simulink model "WindTurbineDrivelineWithVibrations"  (R2023a)
settings: Solver=ode23t  StartTime=0.0  StopTime=scenario.tEnd  MaxStep=2  RelTol=1e-3  AbsTol=1e-3
PreLoadFcn:
  | addpath('Libraries', 'Scripts_Data', 'Images');
model workspace: external: MATLAB File WindTurbineDrivelineWithVibrationsParameters.m (data not in the file)
undefined symbols (not defined in the file): Bampton, Craig, diff, fs, fsCB, m, N, rotor, scenario
libraries: fl_lib x33, nesl_utility x6, simulink x4, sdl_lib x3, slpidlib x1, nesl_utility_internal x1
(part 1 of 2)
CloseFcn:
  | clear fs hModes flex_shaft_mode_props i rotor WindTurbineOut
  | try,close(h1_sscfluids_engine_cooling_system),end
  | clear h1_sscfluids_engine_cooling_system
  | try,close(h2_sscfluids_engine_cooling_system),end
  | clear h2_WindTurbineDrivelineWithVibrations
  | try,close(h3_sscfluids_engine_cooling_system),end
  | clear h3_WindTurbineDrivelineWithVibrations
  | try,close(h4_sscfluids_engine_cooling_system),end
  | clear h4_WindTurbineDrivelineWithVibrations
  | try,close(h5_sscfluids_engine_cooling_system),end
  | clear h5_WindTurbineDrivelineWithVibrations
  | try,close(h6_sscfluids_engine_cooling_system),end
  | clear h6_WindTurbineDrivelineWithVibrations
Description:
  | Wind Turbine Driveline with Vibrations
settings Model: PauseTimes=850  LastModifiedBy=jkluger
settings SolverCC: AutoScaleAbsTol=off  SolverJacobianMethodControl=SparseAnalytical
settings DataIOCC: ReturnWorkspaceOutputsName=WindTurbineOut
settings OptimizationCC: BlockReduction=off  BooleanDataType=off  ReuseModelBlockBuffer=off
settings DebuggingCC: SaveWithParameterizedLinksMsg=none  UnderspecifiedInitializationDetection=Classic  MergeDetectMultiDrivingBlocksExec=none  SignalResolutionControl=TryResolveAllWithWarning
settings HardwareCC: TargetUnknown=on
settings ModelReferenceCC: PropagateSignalLabelsOutOfModel=off
settings SimscapeCC: SimscapeNominalValues="[{\"value\":\"1\",\"unit\":\"1/s\"},   {\"value\":\"1\",\"unit\":\"1\"}, {\"value\":\"1\",\"unit\":\"m/s\"}, {\"value\":\"1\",\"unit\":\"MW\"},{\"value\":\"10\",\"unit\":\"kN\"}, {\"value\":\"1\",\"unit\":\"cm^2\"},{\"value\":\"1\",\"unit\":\"kJ/kg\"},{\"value\":\"1\",\"unit\":\"kN*m\"},{\"value\":\"1\",\"unit\":\"V\"}]"  SimscapeLogType=all  SimscapeLogLimitData=off  SimscapeLogDataHistory=50000

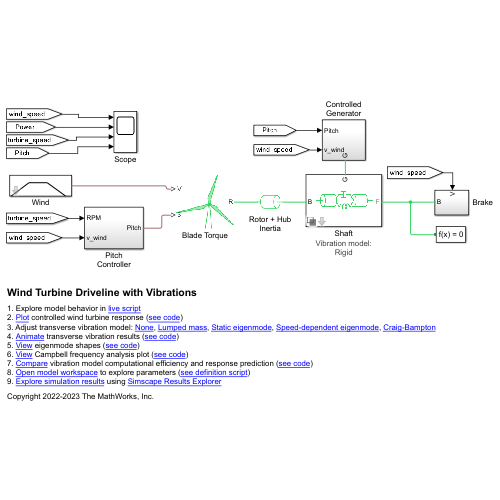
[thumbnail: Simulink's stored preview of the top-level diagram]
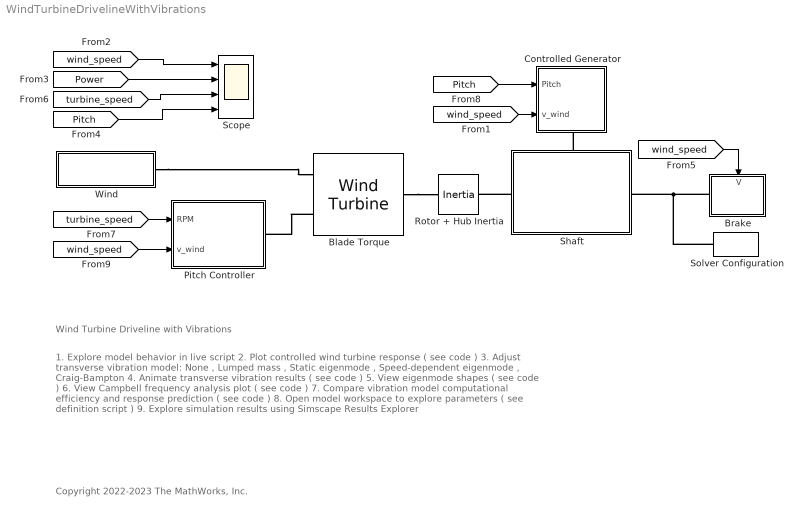
== system WindTurbineDrivelineWithVibrations ==
  note: Wind Turbine Driveline with Vibrations
  note: 1. Explore model behavior in live script
      | 2. Plot controlled wind turbine response ( see code )
      | 3. Adjust transverse vibration model: None , Lumped mass , Static eigenmode , Speed-dependent eigenmode , Craig-Bampton
      | 4. Animate transverse vibration results ( see code )
      | 5. View eigenmode shapes ( see code )
      | 6. View Campbell frequency analysis plot ( see code )
      | 7. Compare vibration model computational efficiency and response prediction ( see code )
      | 8. Open model workspace to explore parameters ( see definition script )
      | 9. Explore simulation results using Simscape Results Explorer
  note: Copyright 2022-2023 The MathWorks, Inc.
  Blade Torque : sdl_lib/Engines & Motors/Wind Turbine  model_thrust=false  R_rotor=rotor.R m  pitch_TLU=rotor.pitch deg  lambda_TLU=rotor.TSR  Cp_TLU=rotor.Cp  Ct_TLU=[0.0000, 0.2451, 0.6740, 0.9616, 1.0000, 0.9882, 0.8430, 0.0002, -0.1341; 0.0016, 0.2541, 0.5942, 0.8582, 0.9561, 0.9754, 0.9599, 0.9092, 0.8669; 0.0027, 0.2705, 0.6113, 0.8503, 0.9339, 0.9407, 0.8993, 0.8016, 0.7239; 0.0054, 0.3215, 0.6475, 0.8205, 0.8482, 0.7727, 0.5565, -0.0450, -0.1171; 0.2035, 0.4335, 0.6485, 0.6348, 0.2129, -0.1684, -0.3701, -0.5712, -0.6681; -0.05 * ones(1, 9)]  rho_air=rotor.rho kg/m^3  model_inertia=false  rotor_inertia=3.5e7 kg*m^2  init_rot_vel=0 rad/s  v_thr=0.01 m/s  w_thr=0.01 rad/s  expose_port_C=0
      settings: InternalSimscapePortConfiguration="{\"Bottom\":[],\"Left\":[{\"id\":\"vWind\",\"label\":\"V\",\"type\":\"input\"},{\"id\":\"pitch\",\"label\":\"β\",\"type\":\"input\"}],\"Right\":[{\"id\":\"R\",\"label\":\"R\",\"type\":\"foundation.mechanical.rotational.rotational\"}],\"Top\":[]}"
  Brake : Subsystem
      settings: PortSchema="{\"entries\":[{\"content\":{\"sides\":[{\"content\":{\"connectorIds\":[\"In1\"]},\"type\":\"ConnectorPlacement.EquallySpacedRectSide\",\"uuid\":\"3f522137-d01e-4a82-a213-9c95e4c48aac\"},{\"content\":{\"connectorIds\":[],\"side\":\"RIGHT\"},\"type\":\"ConnectorPlacement.EquallySpacedRectSide\",\"uuid\":\"7caeb8ed-f130-4046-b756-a57dc180120b\"},{\"content\":{\"connectorIds\":[],\"side\":\"TOP\"},\"type\":\"ConnectorPlacement.EquallySpacedRectSide\",\"uuid\":\"145b1ded-57d7-4746-892b-193b4140ae70\"},{\"content\":{\"connectorIds\":[\"RConn1\"],\"side\":\"BOTTOM\"},\"type\":\"ConnectorPlacement.EquallySpacedRectSide\",\"uuid\":\"4de12456-1f8b-4b22-93b2-a1fd618e5c7f\"}]},\"type\":\"ConnectorPlacement.EquallySpacedConnector\",\"uuid\":\"277f877b-4022-4fd4-aa9a-e474706e0074\"}],\"packageUris\":[\"http://schema.mathworks.com/mf0/Connector/R2020b\"],\"version\":\"1.0\"}"
  Controlled Generator : Subsystem
      settings: PortSchema="{\"entries\":[{\"content\":{\"sides\":[{\"content\":{\"connectorIds\":[\"In1\",\"In2\"]},\"type\":\"ConnectorPlacement.EquallySpacedRectSide\",\"uuid\":\"fea069ae-2c9f-4eba-9b7d-ddf8ed3fb909\"},{\"content\":{\"connectorIds\":[],\"side\":\"RIGHT\"},\"type\":\"ConnectorPlacement.EquallySpacedRectSide\",\"uuid\":\"deeafaeb-3537-4478-830e-60cb40e0f351\"},{\"content\":{\"connectorIds\":[],\"side\":\"TOP\"},\"type\":\"ConnectorPlacement.EquallySpacedRectSide\",\"uuid\":\"3fe5b5b4-073a-4e0c-8561-e9af00445e54\"},{\"content\":{\"connectorIds\":[\"RConn1\"],\"side\":\"BOTTOM\"},\"type\":\"ConnectorPlacement.EquallySpacedRectSide\",\"uuid\":\"d9f3141a-c426-4d0e-bc7d-6e0495890c18\"}]},\"type\":\"ConnectorPlacement.EquallySpacedConnector\",\"uuid\":\"84cb3cad-1caa-4459-9e43-abce1fcb8e5a\"}],\"packageUris\":[\"http://schema.mathworks.com/mf0/Connector/R2020b\"],\"version\":\"1.0\"}"
  Pitch Controller : Subsystem
  Rotor + Hub Inertia : fl_lib/Mechanical/Rotational Elements/Inertia  inertia=rotor.Ip_rotor_hub kg*m^2  num_ports=foundation.enum.numPorts2.two  w_specify=off  w_priority=High  w=0 rad/s  w_nominal_specify=off  w_nominal_unit=rad/s  w_nominal_value=1  t_specify=off  t_priority=None  t=0 N*m  t_nominal_specify=off  t_nominal_unit=N*m  t_nominal_value=1
      settings: InternalSimscapePortConfiguration="{\"Bottom\":[],\"Left\":[{\"id\":\"I\",\"label\":\"\",\"type\":\"foundation.mechanical.rotational.rotational\"}],\"Right\":[{\"id\":\"J\",\"label\":\"\",\"type\":\"foundation.mechanical.rotational.rotational\"}],\"Top\":[]}"
  Scope : Scope  NumInputPorts=4
  Shaft : Subsystem  Variant=on  VariantControlMode=label  VariantControl=Choice  LabelModeActiveChoice=Rigid  mask{vibration_model=Rigid, z_shaft=[0   1   2   3   4   5   6   7   8   9  10], num_modes_eig=24, num_modes_CB=8}
      mask prompts: vibration_model "Vibration model"; z_shaft "Node axial locations"; num_modes_eig "Number of eigenmodes"; num_modes_CB "Number of Craig-Bampton inner modes"
      mask init:
      | % Update num_el_lumped, num_modes_eig, or num_modes_CB
      |     vibration_model= get_param(gcb, 'vibration_model');
      |     set_param(gcb, 'vibration_model', vibration_model);
      settings: PortSchema="{\"entries\":[{\"content\":{\"sides\":[{\"content\":{\"connectorIds\":[\"LConn1\"]},\"type\":\"ConnectorPlacement.EquallySpacedRectSide\",\"uuid\":\"95241633-51a4-426a-b331-3f7eead93793\"},{\"content\":{\"connectorIds\":[\"RConn1\"],\"side\":\"RIGHT\"},\"type\":\"ConnectorPlacement.EquallySpacedRectSide\",\"uuid\":\"d2d9bb5e-ebe8-48ca-b59b-2a6070cc2ba6\"},{\"content\":{\"connectorIds\":[\"LConn2\"],\"side\":\"TOP\"},\"type\":\"ConnectorPlacement.EquallySpacedRectSide\",\"uuid\":\"f68bffd7-2afd-416e-a423-a3b5a698f394\"}]},\"type\":\"ConnectorPlacement.EquallySpacedConnector\",\"uuid\":\"6b30de51-2f46-41e0-9835-7695d3df1ab9\"}],\"packageUris\":[\"http://schema.mathworks.com/mf0/Connector/R2020b\"],\"version\":\"1.0\"}"
      settings: AttributesFormatString=|
      | Vibration model:
      | %<vibration_model>
      mask TypeOptions vibration_model: Rigid | Lumped mass | Static eigenmodes | Speed-dependent eigenmodes | Craig-Bampton
      mask Callback vibration_model:
      | vibration_model= get_param(gcb, 'vibration_model');
      |     mdlWks = get_param(bdroot,'ModelWorkspace');
      |     solver= getVariable(mdlWks, 'solver');
      |     fs= getVariable(mdlWks, 'fs');
      |     if strcmp(vibration_model, 'Rigid')
      |         paramVisibility= {'on','off', 'off', 'off'};
      |         set_param(bdroot, 'SimscapeNominalValues', solver.SimscapeNominalValues.rigid);
      |     elseif strcmp(vibration_model, 'Lumped mass')
      |         paramVisibility= {'on', 'on', 'off', 'off'};
      |         set_param(bdroot, 'SimscapeNominalValues', solver.SimscapeNominalValues.lumped_mass);
      |         z_shaft= eval(get_param(gcb, 'z_shaft'));
      |         fs.z_shaft= z_shaft;
      |         mdlWks.assignin('fs', fs)
      |     elseif strcmp(vibration_model, 'Static eigenmodes')
      |         paramVisibility= {'on', 'off', 'on', 'off'};
      |         set_param(bdroot, 'SimscapeNominalValues', solver.SimscapeNominalValues.static_eig);
      |         num_modes_eig= eval(get_param(gcb, 'num_modes_eig'));
      |         fs.num_modes= num_modes_eig;
      |         mdlWks.assignin('fs', fs);
      |     elseif strcmp(vibration_model, 'Speed-dependent eigenmodes')
      |         paramVisibility= {'on', 'off', 'on', 'off'};
      |         set_param(bdroot, 'SimscapeNominalValues', solver.SimscapeNominalValues.speed_dep_eig);
      |         num_modes_eig= eval(get_param(gcb, 'num_modes_eig'));
      |         fs.num_modes= num_modes_eig;
      |         mdlWks.assignin('fs', fs);
      |     else % vibration_model == 'Craig-Bampton'
      |         paramVisibility= {'on', 'off', 'off', 'on'};
      |         set_param(bdroot, 'SimscapeNominalValues', solver.SimscapeNominalValues.CB);
      |         fs.ne_Lumped= 50;
      |         fs.z_shaft= linspace(0, fs.length_shaft, fs.ne_Lumped);
      |         fsCB= fs;
      |         fsCB.num_modes= eval(get_param(gcb, 'num_modes_CB'));
      |         fsCB= WindTurbineDrivelineWithVibrationsCraigBamptonReduction(fsCB);
      |         mdlWks.assignin('fsCB', fsCB)
      |     end
      |     assignin('base', 'fs', fs);
      |     set_param(gcb,'MaskVisibilities',paramVisibility);
      |     set_param(gcb,'OverrideUsingVariant', vibration_model);
      mask Callback z_shaft:
      | mdlWks = get_param(bdroot,'ModelWorkspace');
      |     fs= getVariable(mdlWks, 'fs');
      |     z_shaft= eval(get_param(gcb, 'z_shaft'));
      |     fs.z_shaft= z_shaft;
      |     mdlWks = get_param(bdroot,'ModelWorkspace');
      |     mdlWks.assignin('fs', fs)
      |     assignin('base', 'fs', fs);
      mask Callback num_modes_eig:
      | mdlWks = get_param(bdroot,'ModelWorkspace');
      |     fs= getVariable(mdlWks, 'fs');
      |     num_modes_eig= eval(get_param(gcb, 'num_modes_eig'));
      |     fs.num_modes= num_modes_eig;
      |     mdlWks.assignin('fs', fs);
      |     assignin('base', 'fs', fs);
      mask Callback num_modes_CB:
      | mdlWks = get_param(bdroot,'ModelWorkspace');
      |     fs= getVariable(mdlWks, 'fs');
      |     fs.ne_Lumped= 50;
      |     fs.z_shaft= linspace(0, fs.length_shaft, fs.ne_Lumped);
      |     fsCB= fs;
      |     fsCB.num_modes= eval(get_param(gcb, 'num_modes_CB'));
      |     fsCB= WindTurbineDrivelineWithVibrationsCraigBamptonReduction(fsCB);
      |     mdlWks.assignin('fsCB', fsCB)
      |     assignin('base', 'fs', fs);
      mask DialogControl Shaft Prompt: Shaft
      mask DialogControl DescTextVar Prompt: This block models the transverse vibrations of a rotating shaft.
      mask Display: image('WindTurbineDrivelineWithVibrationsIcon.jpg');
  Solver Configuration : nesl_utility_internal/Solver Configuration  PhysicalDomain=network_engine_domain  SubClassName=solver  LeftPortType=input  RightPortType=generic  Tones=[]  Harmonics=[]  SimulateNoise=off  Profile=off  UseLocalSampling=off  EnableSwitchedLinearOptims=on  FrequencyDomain=off  UseCCode=off  RelTol=0.001  AbsTol=1e-06  MinStep=1e-09  ToWorkspace=off  RevertToSquareIcSolve=off  NumHomotopyIterations=100  PhasorMode=off  PhasorModeNumHarmonics=1  ConsistencySolver=NEWTON_XTOL_AFTER_FTOL  IndexReductionMethod=DerivativeReplacement  DoDC=off  ResidualTolerance=1e-9  ConsistencyTolSource=GLOBAL  ConsistencyAbsTol=0.001  ConsistencyRelTol=0.001  ConsistencyTolFactor=0.001  UseLocalSolver=off  LocalSolverChoice=NE_TRAPEZOIDAL_ADVANCER  ResolveIndetEquations=on  FunctionEvalNumThread=1  LocalSolverSampleTime=.002  DoFixedCost=off  MaxNonlinIter=3  MaxModeIter=2  ComputeImpulses=off  ImpulseIterations=2  LinearAlgebra=auto  LinearAlgebraNumThread=0  EquationFormulation=NE_TIME_EF  DelaysMemoryBudget=1024  AutomaticFiltering=on  FilteringTimeConstant=0.001  PartitionStorageMethod=AS_NEEDED  PartitionMemoryBudget=1024  PartitionMethod=FAST
  Wind : Subsystem  VariantControl=Ramp  mask{time=scenario.wind.Time, values=scenario.wind.Values}
      mask prompts: time "Time (s)"; values "Wind speed (m/s)"
      mask Display:
      | plot(0, 0)
      | plot(30, 30)
      | mdlWks = get_param(bdroot,'ModelWorkspace');
      | Time= evalin(mdlWks, get_param(gcb, 'time'));
      | windSpeed= evalin(mdlWks, get_param(gcb, 'values'));
      | plot(Time, windSpeed);
  wires:
  [wind_speed] -> Scope/1
  [turbine_speed] -> Scope/3
  [Power] -> Scope/2
  [Pitch] -> Scope/4
  [turbine_speed] -> Pitch Controller/1(RPM)
  [Pitch] -> Controlled Generator/1(Pitch)
  [wind_speed] -> Controlled Generator/2(v_wind)
  [wind_speed] -> Brake/1(V)
  [wind_speed] -> Pitch Controller/2(v_wind)
  connections:
  Brake/RConn1 -- Solver Configuration/RConn1 -- Shaft/RConn1
  Blade Torque/LConn2 -- Pitch Controller/RConn1
  Wind/RConn1 -- Blade Torque/LConn1
  Shaft/LConn1 -- Rotor + Hub Inertia/LConn1
  Shaft/LConn2 -- Controlled Generator/RConn1
  Blade Torque/RConn1 -- Rotor + Hub Inertia/RConn1

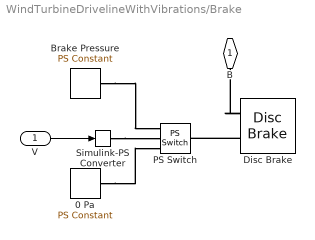
== system WindTurbineDrivelineWithVibrations/Brake ==
  V : Inport
  0 Pa : fl_lib/Physical Signals/Sources/PS Constant  constant=0 Pa
  Brake Pressure : fl_lib/Physical Signals/Sources/PS Constant  constant=10^9 Pa
  Disc Brake : sdl_lib/Brakes & Detents/Rotational/Disc Brake  r_mean=rotor.brake.radius m  bore=0.1*rotor.brake.radius m  n_pads=2  thermal_port=simscape.enum.thermaleffects.omit  mu_static=0.9  mu_coulomb=0.7  temperature_TLU=[280, 300, 320] K  mu_static_TLU=[.9, .8, .7]  mu_coulomb_TLU=[.8, .7, .6]  brkwy_vel=0.1 rad/s  visc_coef=0 N*m/(rad/s)  enable_faults=simscape.enum.onoff.off  faulted_pressure=0 bar  external_fault=simscape.enum.onoff.off  temporal_fault=simscape.enum.onoff.off  fault_time=5 s  report_fault=simscape.enum.assert.action.none  thermal_mass=50 kJ/K  temperature_specify=off  temperature_priority=High  temperature=300 K  temperature_nominal_specify=off  temperature_nominal_unit=K  temperature_nominal_value=1
  PS Switch : fl_lib/Physical Signals/Nonlinear Operators/PS Switch  Threshold=rotor.max_wind_speed m/s
      settings: InternalSimscapePortConfiguration="{\"Bottom\":[],\"Left\":[{\"id\":\"I1\",\"label\":\"\",\"type\":\"input\"},{\"id\":\"I2\",\"label\":\"\",\"type\":\"input\"},{\"id\":\"I3\",\"label\":\"\",\"type\":\"input\"}],\"Right\":[{\"id\":\"O\",\"label\":\"\",\"type\":\"output\"}],\"Top\":[]}"
  Simulink-PS Converter : nesl_utility/Simulink-PS Converter  PhysicalDomain=network_engine_domain  SubClassName=ps_input  LeftPortType=input  RightPortType=output  PseudoPeriodic=off  Frequencies=[]  NoiseDistribution=none  NoiseParameters=[]  Unit=m/s  AffineConversion=off  FilteringAndDerivatives=provide  SimscapeFilterOrder=1  InputFilterTimeConstant=0.001  UdotUserProvided=0
  B : PMIOPort  Side=Right
  wires:
  V/1 -> Simulink-PS Converter/1
  connections:
  Disc Brake/LConn2 -- B/RConn1
  Disc Brake/LConn1 -- PS Switch/RConn1
  Simulink-PS Converter/RConn1 -- PS Switch/LConn2
  0 Pa/RConn1 -- PS Switch/LConn3
  Brake Pressure/RConn1 -- PS Switch/LConn1

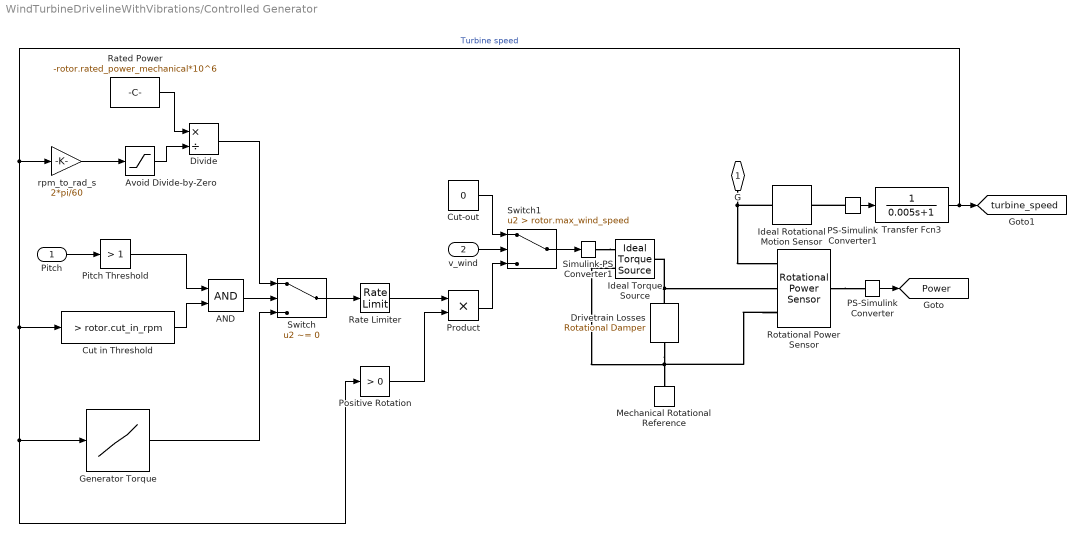
== system WindTurbineDrivelineWithVibrations/Controlled Generator ==
  Pitch : Inport
  v_wind : Inport  Port=2
  AND : Logic  AllPortsSameDT=off  OutDataTypeStr=boolean
  Avoid Divide-by-Zero : Saturate  UpperLimit=inf  LowerLimit=0.01  ZeroCross=off
  Cut in Threshold : simulink/Logic and Bit Operations/Compare To Constant  relop=>  const=rotor.cut_in_rpm  OutDataTypeStr=boolean
  Cut-out : Constant  Value=0
  Divide : Product  Inputs=*/
  Drivetrain Losses : fl_lib/Mechanical/Rotational Elements/Rotational Damper  D=rotor.drivetrain_losses_damping N*m/(rad/s)  w_specify=off  w_priority=None  w=0 rad/s  w_nominal_specify=off  w_nominal_unit=rad/s  w_nominal_value=1  t_specify=off  t_priority=None  t=0 N*m  t_nominal_specify=off  t_nominal_unit=N*m  t_nominal_value=1
  Generator Torque : Lookup_n-D  NumberOfTableDimensions=1  BreakpointsForDimension1=rotor.generator_speed_TLU % rpm  Table=-rotor.generator_torque_TLU % N*m  ExtrapMethod=Clip  UseLastTableValue=on  InternalRulePriority=Speed  RndMeth=Simplest
  Ideal Torque Source : fl_lib/Mechanical/Mechanical Sources/Ideal Torque Source
  Ideal Rotational Motion Sensor : fl_lib/Mechanical/Mechanical Sensors/Ideal Rotational Motion Sensor  reference=foundation.enum.MeasurementReference.absolute  acceleration_port=false  velocity_port=true  position_port=false  wrap_angle=simscape.enum.onoff.off  offset=0 rad
      settings: InternalSimscapePortConfiguration="{\"Bottom\":[],\"Left\":[{\"id\":\"R\",\"label\":\"R\",\"type\":\"foundation.mechanical.rotational.rotational\"}],\"Right\":[{\"id\":\"W\",\"label\":\"W\",\"type\":\"output\"}],\"Top\":[]}"
  Mechanical Rotational Reference : fl_lib/Mechanical/Rotational Elements/Mechanical Rotational Reference
  PS-Simulink Converter : nesl_utility/PS-Simulink Converter  PhysicalDomain=network_engine_domain  SubClassName=ps_output  LeftPortType=input  RightPortType=output  PseudoPeriodic=off  Frequencies=[]  VectorFormat=1-D array  Unit=MW  AffineConversion=off
  PS-Simulink Converter1 : nesl_utility/PS-Simulink Converter  PhysicalDomain=network_engine_domain  SubClassName=ps_output  LeftPortType=input  RightPortType=output  PseudoPeriodic=off  Frequencies=[]  VectorFormat=1-D array  Unit=rpm  AffineConversion=off
  Pitch Threshold : simulink/Logic and Bit Operations/Compare To Constant  relop=>  const=1  OutDataTypeStr=boolean  ZeroCross=off
  Positive Rotation : simulink/Logic and Bit Operations/Compare To Constant  relop=>  const=0  OutDataTypeStr=boolean  ZeroCross=off
  Product : Product
  Rate Limiter : RateLimiter  RisingSlewLimit=rotor.torque_rated*5  FallingSlewLimit=-rotor.torque_rated*5  SampleTimeMode=inherited
  Rated Power : Constant  Value=-rotor.rated_power_mechanical*10^6
  Rotational Power Sensor : sdl_lib/Sensors/Rotational Power Sensor  measurement_type=sdl.enum.rotationalPowerSensorType.instantaneous  averaging_period=1 s  max_frequency=1000 Hz  max_speed=1000 rpm
      settings: InternalSimscapePortConfiguration="{\"Bottom\":[],\"Left\":[{\"id\":\"S\",\"label\":\"S\",\"type\":\"foundation.mechanical.rotational.rotational\"},{\"id\":\"R\",\"label\":\"R\",\"type\":\"foundation.mechanical.rotational.rotational\"},{\"id\":\"C\",\"label\":\"C\",\"type\":\"foundation.mechanical.rotational.rotational\"}],\"Right\":[{\"id\":\"P\",\"label\":\"P\",\"type\":\"output\"}],\"Top\":[]}"
  Simulink-PS Converter1 : nesl_utility/Simulink-PS Converter  PhysicalDomain=network_engine_domain  SubClassName=ps_input  LeftPortType=input  RightPortType=output  PseudoPeriodic=off  Frequencies=[]  NoiseDistribution=none  NoiseParameters=[]  Unit=N*m  AffineConversion=off  FilteringAndDerivatives=provide  SimscapeFilterOrder=1  InputFilterTimeConstant=0.001  UdotUserProvided=0
  Switch : Switch  Criteria=u2 ~= 0  Threshold=1  SaturateOnIntegerOverflow=off  InputSameDT=off
  Switch1 : Switch  Criteria=u2 > Threshold  Threshold=rotor.max_wind_speed  SaturateOnIntegerOverflow=off  InputSameDT=off
  Transfer Fcn3 : TransferFcn  Denominator=[0.005 1]
  rpm_to_rad_s : Gain  Gain=2*pi/60
  G : PMIOPort  Side=Right
  tag scope: Power=global, turbine_speed=global
  wires:
  PS-Simulink Converter/1 -> [Power]
  Transfer Fcn3/1 -> [turbine_speed], Generator Torque/1, Positive Rotation/1, Cut in Threshold/1, rpm_to_rad_s/1  "Turbine speed"
  Switch/1 -> Rate Limiter/1
  Generator Torque/1 -> Switch/3
  Rated Power/1 -> Divide/1
  Avoid Divide-by-Zero/1 -> Divide/2
  Divide/1 -> Switch/1
  rpm_to_rad_s/1 -> Avoid Divide-by-Zero/1
  PS-Simulink Converter1/1 -> Transfer Fcn3/1
  v_wind/1 -> Switch1/2
  Cut-out/1 -> Switch1/1
  Switch1/1 -> Simulink-PS Converter1/1
  Pitch/1 -> Pitch Threshold/1
  Pitch Threshold/1 -> AND/1
  Cut in Threshold/1 -> AND/2
  AND/1 -> Switch/2
  Rate Limiter/1 -> Product/1
  Positive Rotation/1 -> Product/2
  Product/1 -> Switch1/3
  connections:
  Drivetrain Losses/LConn1 -- Rotational Power Sensor/LConn2 -- Ideal Torque Source/LConn1
  Rotational Power Sensor/LConn3 -- Drivetrain Losses/RConn1 -- Ideal Torque Source/RConn2 -- Mechanical Rotational Reference/LConn1
  Rotational Power Sensor/RConn1 -- PS-Simulink Converter/LConn1
  G/RConn1 -- Ideal Rotational Motion Sensor/LConn1 -- Rotational Power Sensor/LConn1
  Simulink-PS Converter1/RConn1 -- Ideal Torque Source/RConn1
  PS-Simulink Converter1/LConn1 -- Ideal Rotational Motion Sensor/RConn1

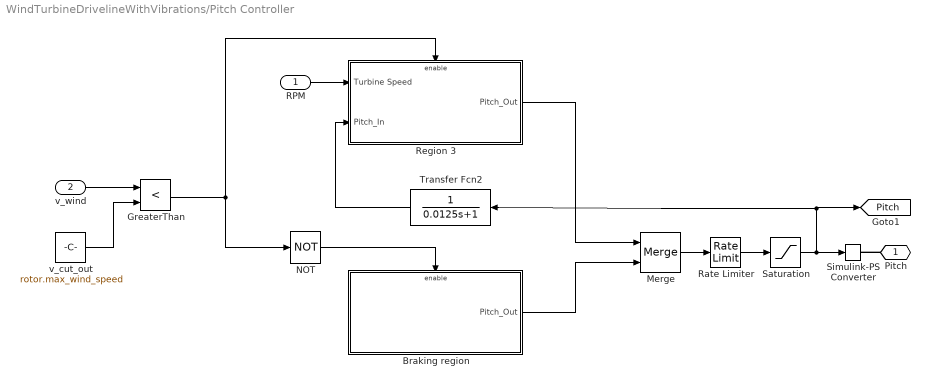
== system WindTurbineDrivelineWithVibrations/Pitch Controller ==
  RPM : Inport
  v_wind : Inport  Port=2
  Braking region : Subsystem
  GreaterThan : RelationalOperator  Operator=<  OutDataTypeStr=boolean  ZeroCross=off  RndMeth=Simplest  InputSameDT=off
  Merge : Merge
  NOT : Logic  Operator=NOT  AllPortsSameDT=off  OutDataTypeStr=boolean
  Rate Limiter : RateLimiter  RisingSlewLimit=8  FallingSlewLimit=-8  SampleTimeMode=inherited
  Region 3 : Subsystem
  Saturation : Saturate  UpperLimit=90  LowerLimit=0  ZeroCross=off
  Simulink-PS Converter : nesl_utility/Simulink-PS Converter  PhysicalDomain=network_engine_domain  SubClassName=ps_input  LeftPortType=input  RightPortType=output  PseudoPeriodic=off  Frequencies=[]  NoiseDistribution=none  NoiseParameters=[]  Unit=deg  AffineConversion=off  FilteringAndDerivatives=provide  SimscapeFilterOrder=1  InputFilterTimeConstant=0.001  UdotUserProvided=0
  Transfer Fcn2 : TransferFcn  Denominator=[0.0125 1]
  v_cut_out : Constant  Value=rotor.max_wind_speed
  Pitch : PMIOPort  Side=Right
  tag scope: Pitch=global
  wires:
  RPM/1 -> Region 3/1(Turbine Speed)
  Transfer Fcn2/1 -> Region 3/2(Pitch_In)
  Saturation/1 -> Transfer Fcn2/1, [Pitch], Simulink-PS Converter/1
  v_wind/1 -> GreaterThan/1
  v_cut_out/1 -> GreaterThan/2
  GreaterThan/1 -> NOT/1, Region 3/Enable
  Region 3/1(Pitch_Out) -> Merge/1
  Braking region/1(Pitch_Out) -> Merge/2
  Rate Limiter/1 -> Saturation/1
  Merge/1 -> Rate Limiter/1
  NOT/1 -> Braking region/Enable
  connections:
  Pitch/RConn1 -- Simulink-PS Converter/RConn1

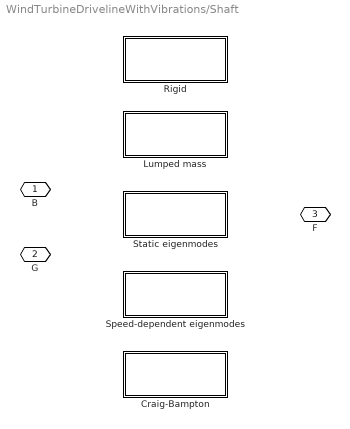
== system WindTurbineDrivelineWithVibrations/Shaft ==
  Craig-Bampton : Subsystem  VariantControl=Craig-Bampton
  Lumped mass : Subsystem  VariantControl=Lumped mass
  Rigid : Subsystem  VariantControl=Rigid
  Speed-dependent eigenmodes : Subsystem  VariantControl=Speed-dependent eigenmodes
  Static eigenmodes : Subsystem  VariantControl=Static eigenmodes
  B : PMIOPort  Side=Left
  G : PMIOPort  Port=2  Side=Left
  F : PMIOPort  Port=3  Side=Right

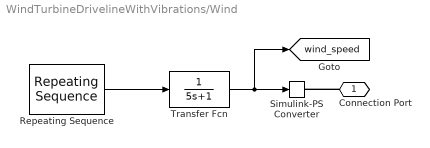
== system WindTurbineDrivelineWithVibrations/Wind ==
  Repeating Sequence : simulink/Sources/Repeating Sequence  rep_seq_t=time  rep_seq_y=values
  Simulink-PS Converter : nesl_utility/Simulink-PS Converter  PhysicalDomain=network_engine_domain  SubClassName=ps_input  LeftPortType=input  RightPortType=output  PseudoPeriodic=off  Frequencies=[]  NoiseDistribution=none  NoiseParameters=[]  Unit=m/s  AffineConversion=off  FilteringAndDerivatives=provide  SimscapeFilterOrder=1  InputFilterTimeConstant=0.001  UdotUserProvided=0
  Transfer Fcn : TransferFcn  Denominator=[5 1]
  Connection Port : PMIOPort  Side=Right
  tag scope: wind_speed=global
  wires:
  Repeating Sequence/1 -> Transfer Fcn/1
  Transfer Fcn/1 -> [wind_speed], Simulink-PS Converter/1
  connections:
  Connection Port/RConn1 -- Simulink-PS Converter/RConn1

== system WindTurbineDrivelineWithVibrations/Pitch Controller/Braking region ==
  Enable : EnablePort
  Feather Blades : Constant  Value=90
  Pitch_Out : Outport  InitialOutput=90
  wires:
  Feather Blades/1 -> Pitch_Out/1

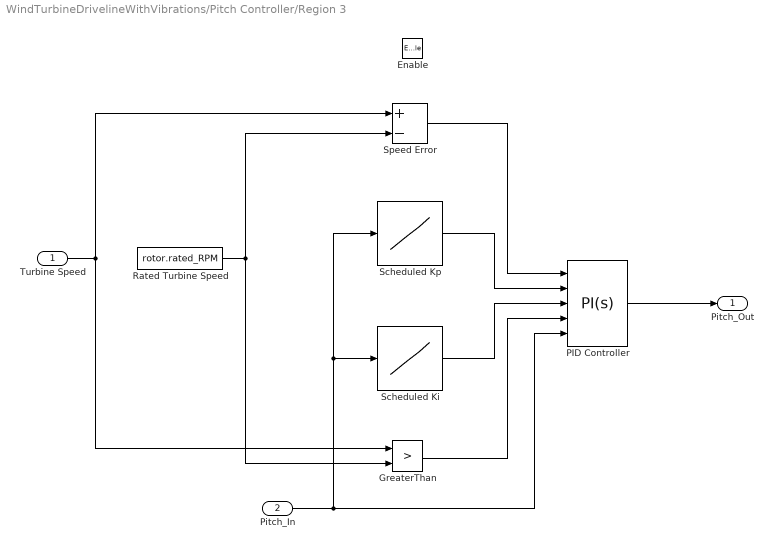
== system WindTurbineDrivelineWithVibrations/Pitch Controller/Region 3 ==
  Turbine Speed : Inport
  Pitch_In : Inport  Port=2
  Enable : EnablePort  StatesWhenEnabling=reset
  GreaterThan : RelationalOperator  Operator=>  OutDataTypeStr=boolean  ZeroCross=off  RndMeth=Simplest  InputSameDT=off
  PID Controller : slpidlib/PID Controller  Controller=PI  Form=Parallel  TimeDomain=Continuous-time  UseExternalTs=off  SampleTime=-1  IntegratorMethod=Forward Euler  FilterMethod=Forward Euler  ControllerParametersSource=external  P=0.12  I=8  UseKiTs=off  D=0  N=100  UseFilter=on  TunerSelectOption=Transfer Function Based (PID Tuner App)  ZeroCross=off  InitialConditionSource=external  InitialConditionForIntegrator=rotor.pitch(1)  InitialConditionForFilter=0  DifferentiatorICPrevScaledInput=0  ExternalReset=either  TrackingMode=off  Kt=1  LimitOutput=on  SatLimitsSource=internal  UpperSaturationLimit=90  LowerSaturationLimit=0  LinearizeAsGain=on  AntiWindupMode=none  Kb=1  LimitIntegrator=off  UpperIntegratorSaturationLimit=inf  LowerIntegratorSaturationLimit=-inf  POutMin=[]  POutMax=[]  IOutMin=[]  IOutMax=[]  DOutMin=[]  DOutMax=[]  NOutMin=[]  NOutMax=[]  SumOutMin=[]  SumOutMax=[]  SaturationOutMin=[]  SaturationOutMax=[]  PParamMin=[]  PParamMax=[]  IParamMin=[]  IParamMax=[]  DParamMin=[]  DParamMax=[]  NParamMin=[]  NParamMax=[]  KbParamMin=[]  KbParamMax=[]  KtParamMin=[]  KtParamMax=[]  KbOutMin=[]  KbOutMax=[]  KtOutMin=[]  KtOutMax=[]  IntegratorOutMin=[]  IntegratorOutMax=[]  FilterOutMin=[]  FilterOutMax=[]  SumI1OutMin=[]  SumI1OutMax=[]  SumI2OutMin=[]  SumI2OutMax=[]  SumI3OutMin=[]  SumI3OutMax=[]  SumI4OutMin=[]  SumI4OutMax=[]  SumDOutMin=[]  SumDOutMax=[]  DifferentiatorOutMin=[]  DifferentiatorOutMax=[]  FilterDiffOutCoefMin=[]  FilterDiffOutCoefMax=[]  ReciprocalOutMin=[]  ReciprocalOutMax=[]  SumDenOutMin=[]  SumDenOutMax=[]  SumNumOutMin=[]  SumNumOutMax=[]  DivideOutMin=[]  DivideOutMax=[]  UdiffTsProdOutMin=[]  UdiffTsProdOutMax=[]  NTsProdOutMin=[]  NTsProdOutMax=[]  UintegralTsProdOutMin=[]  UintegralTsProdOutMax=[]  UngainTsProdOutMin=[]  UngainTsProdOutMax=[]  ClampingZeroOutDataTypeStr=Inherit: Inherit via back propagation  ClampingZeroOutMin=[]  ClampingZeroOutMax=[]  FilterDenConstantOutDataTypeStr=Inherit: Inherit via back propagation  FilterDenConstantOutMin=[]  FilterDenConstantOutMax=[]  PCopyOutDataTypeStr=Inherit: Inherit via back propagation  PCopyOutMin=[]  PCopyOutMax=[]  NCopyOutDataTypeStr=Inherit: Inherit via back propagation  NCopyOutMin=[]  NCopyOutMax=[]  IntegratorContinuousStateAttributes=''  IntegratorStateMustResolveToSignalObject=off  IntegratorRTWStateStorageClass=Auto  FilterContinuousStateAttributes=''  FilterStateMustResolveToSignalObject=off  FilterRTWStateStorageClass=Auto  ParallelPVariant=ExternalParameters  IdealPVariant=Disabled  IVariant=ExternalParameters  DVariant=Disabled  IntegratorVariant=Continuous  SatVariant=Enabled  AWVariant=Passthrough  PCopyVariant=Disabled  TRVariant=Disabled  FdbkBlocksVariant=Forward  IdealPFdbkVariant=Disabled  SatFdbkVariant=Disabled  DerivativeFilterVariant=Disabled  NVariant=Disabled  NCopyVariant=Disabled_SignalSpec  FilterICVariant=Disabled  IntegratorICVariant=ExternalICs  ExternalResetVariant=ExternalReset  TRSumVariant=Passthrough  SumFdbkVariant=Disabled  SumVariant=Sum_PI  TsampFilterVariant=InternalTs  TsampNgainVariant=Passthrough  TsampIntegralVariant=Disabled_SignalSpec  ExternalSaturationOutDataTypeStr=Inherit: Same as second input
  Rated Turbine Speed : Constant  Value=rotor.rated_RPM
  Scheduled Ki : Lookup_n-D  NumberOfTableDimensions=1  BreakpointsForDimension1=rotor.pitch_TLU  Table=rotor.pitch_Ki_TLU  InternalRulePriority=Speed  RndMeth=Simplest
  Scheduled Kp : Lookup_n-D  NumberOfTableDimensions=1  BreakpointsForDimension1=rotor.pitch_TLU  Table=rotor.pitch_Kp_TLU  InternalRulePriority=Speed  RndMeth=Simplest
  Speed Error : Sum  Inputs=+-
  Pitch_Out : Outport
  wires:
  Pitch_In/1 -> Scheduled Ki/1, Scheduled Kp/1, PID Controller/5
  Scheduled Kp/1 -> PID Controller/2
  Speed Error/1 -> PID Controller/1
  Scheduled Ki/1 -> PID Controller/3
  Turbine Speed/1 -> GreaterThan/1, Speed Error/1
  Rated Turbine Speed/1 -> GreaterThan/2, Speed Error/2
  GreaterThan/1 -> PID Controller/4
  PID Controller/1 -> Pitch_Out/1

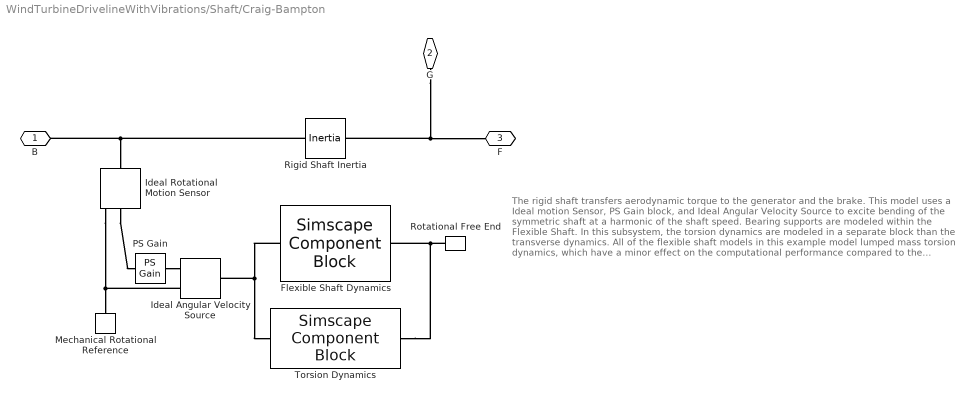
== system WindTurbineDrivelineWithVibrations/Shaft/Craig-Bampton ==
  note: The rigid shaft transfers aerodynamic torque to the generator and the brake.
      |
      | This model uses a Ideal motion Sensor, PS Gain block, and Ideal Angular Velocity Source to excite bending of the symmetric shaft at a harmonic of the shaft speed. Bearing supports are modeled within the Flexible Shaft.
      |
      | In this subsystem, the torsion dynamics are modeled in a separate block than the transverse dynamics. All of the flexible shaft models in this example model lumped mass torsion dynamics, which have a minor effect on the computational performance compared to the transverse dynamics.
  Flexible Shaft Dynamics : SimscapeComponentBlock  SourceFile=WindTurbineDrivelineWithVibrationsFlexibleShaftCB  ComponentPath=WindTurbineDrivelineWithVibrationsFlexibleShaftCB  ComponentVariants="[\"WindTurbineDrivelineWithVibrationsFlexibleShaftCB\"]"  ComponentVariantNames="[\"WindTurbineDrivelineWithVibrationsFlexibleShaftCB\"]"  ClassName=WindTurbineDrivelineWithVibrationsFlexibleShaftCB  SchemaVersion=1  M=fsCB.M  normM=fsCB.normM  G=fsCB.G  K=fsCB.K 1/s^2  alpha=fsCB.a_damp 1/s  beta=fsCB.b_damp s  ForceMagnitude=fsCB.F  num_primary_nodes=fsCB.num_primary_nodes  eta_nominal_value=solver.SimscapeNominalValues.fsCB.mode_displacements  etaDer_nominal_value=SimscapeNominalValues.fsCB.mode_velocities  support_node=fsCB.support_nodes  bearing_speed=fs.bearing_speed rad/s  K_supportB1=fs.bearing.K N/m  D_supportB1=fs.bearing.D N*s/m  Krot_supportB1=fs.bearing.k_rot N*m/rad  Drot_supportB1=fs.bearing.d_rot N*m*s/rad  K_supportI1=fs.bearing.K N/m  D_supportI1=fs.bearing.D N*s/m  Krot_supportI1=fs.bearing.k_rot N*m/rad  Drot_supportI1=fs.bearing.d_rot N*m*s/rad  K_supportI2=fs.bearing.K N/m  D_supportI2=fs.bearing.D N*s/m  Krot_supportI2=fs.bearing.k_rot N*m/rad  Drot_supportI2=fs.bearing.d_rot N*m*s/rad  K_supportI3=fs.bearing.k_trans_speed_Free N/m  D_supportI3=fs.bearing.d_trans_speed_Free N*s/m  Krot_supportI3=fs.bearing.k_rot_Free N*m/rad  Drot_supportI3=fs.bearing.d_rot_Free N*m*s/rad  K_supportF1=fs.bearing.K N/m  D_supportF1=fs.bearing.D N*s/m  Krot_supportF1=fs.bearing.k_rot N*m/rad  Drot_supportF1=fs.bearing.d_rot N*m*s/rad  t_specify=off  t_priority=None  t=0 N*m  t_nominal_specify=off  t_nominal_unit=N*m  t_nominal_value=1  w_specify=off  w_priority=None  w=0 rad/s  w_nominal_specify=off  w_nominal_unit=rad/s  w_nominal_value=1  wDer_specify=off  wDer_priority=None  wDer=0 rad/s^2  wDer_nominal_specify=off  wDer_nominal_unit=rad/s^2  wDer_nominal_value=1  phi_specify=off  phi_priority=None  phi=0 rad  phi_nominal_specify=off  phi_nominal_unit=rad  phi_nominal_value=1  Bfx_specify=off  Bfx_priority=None  Bfx=0 N  Bfx_nominal_specify=off  Bfx_nominal_unit=N  Bfx_nominal_value=1  Bfy_specify=off  Bfy_priority=None  Bfy=0 N  Bfy_nominal_specify=off  Bfy_nominal_unit=N  Bfy_nominal_value=1  BTx_specify=off  BTx_priority=None  BTx=0 N*m  BTx_nominal_specify=off  BTx_nominal_unit=N*m  BTx_nominal_value=1  BTy_specify=off  BTy_priority=None  BTy=0 N*m  BTy_nominal_specify=off  BTy_nominal_unit=N*m  BTy_nominal_value=1
      settings: CopyFcn=simscape.engine.sli.internal.componentblockcallback(gcbh,'COPY')  PreCopyFcn=simscape.engine.sli.internal.componentblockcallback(gcbh,'PRECOPY')  PreDeleteFcn=simscape.engine.sli.internal.componentblockcallback(gcbh,'PREDELETE')  InternalSimscapePortConfiguration="{\"Bottom\":[],\"Left\":[{\"id\":\"B\",\"label\":\"B\",\"type\":\"foundation.mechanical.rotational.rotational\"}],\"Right\":[{\"id\":\"F\",\"label\":\"F\",\"type\":\"foundation.mechanical.rotational.rotational\"}],\"Top\":[]}"
      mask Type: Craig-Bampton Flexible Shaft
  Ideal Angular Velocity Source : fl_lib/Mechanical/Mechanical Sources/Ideal Angular Velocity Source
  Ideal Rotational Motion Sensor : fl_lib/Mechanical/Mechanical Sensors/Ideal Rotational Motion Sensor  reference=foundation.enum.MeasurementReference.difference  acceleration_port=false  velocity_port=true  position_port=true  wrap_angle=false  offset=0 rad
  Mechanical Rotational Reference : fl_lib/Mechanical/Rotational Elements/Mechanical Rotational Reference
  PS Gain : fl_lib/Physical Signals/Functions/PS Gain  gain=fs.excitationPoles
  Rigid Shaft Inertia : fl_lib/Mechanical/Rotational Elements/Inertia  inertia=fs.Ip_total kg*m^2  num_ports=foundation.enum.numPorts2.two  w_specify=off  w_priority=High  w=0 rad/s  w_nominal_specify=off  w_nominal_unit=rad/s  w_nominal_value=1  t_specify=off  t_priority=None  t=0 N*m  t_nominal_specify=off  t_nominal_unit=N*m  t_nominal_value=1
      settings: InternalSimscapePortConfiguration="{\"Bottom\":[],\"Left\":[{\"id\":\"I\",\"label\":\"\",\"type\":\"foundation.mechanical.rotational.rotational\"}],\"Right\":[{\"id\":\"J\",\"label\":\"\",\"type\":\"foundation.mechanical.rotational.rotational\"}],\"Top\":[]}"
  Rotational Free End : fl_lib/Mechanical/Rotational Elements/Rotational Free End  w_specify=off  w_priority=None  w=0 rad/s  w_nominal_specify=off  w_nominal_unit=rad/s  w_nominal_value=1
  Torsion Dynamics : SimscapeComponentBlock  SourceFile=sdl.couplings.flexible_shaft  ComponentPath=sdl.couplings.flexible_shaft  ComponentVariants="[\"sdl.couplings.flexible_shaft\"]"  ComponentVariantNames="[\"flexible_shaft\"]"  ClassName=flexible_shaft  SchemaVersion=1  modelTorsion=true  modelTransverse=false  n_segments=1  parameterization=sdl.enum.shaftParameterization.MaterialPropertiesVaried  length=fs.length_shaft m  lengths=diff(fs.z_shaft) m  shaft_stiffness=2e5 N*m/rad  shaft_inertia=0.02 kg*m^2  shaft_stiffnesses=[400000, 200000, 100000] N*m/rad  shaft_inertias=[.025, .02, .015] kg*m^2  eiIN=5e5 Pa*m^4  rhoaIN=19 kg/m  eiINs=[600000, 500000, 400000] Pa*m^4  rhoaINs=[20, 19, 18] kg/m  density=fs.material_density kg/m^3  shear_modulus=fs.shear_modulus Pa  elastic_modulus=fs.elastic_modulus Pa  shaft_construction=sdl.enum.shaftConstruction.annular  diameter_outer=fs.diameters_outer(1) m  diameter_inner=fs.diameters_inner(1) m  diameter_outers=interp1(fs.z_TLU, fs.diameters_outer_TLU, fs.z_shaft(2:end)) m  diameter_inners=interp1(fs.z_TLU, fs.diameters_inner_TLU, fs.z_shaft(2:end)) m  damping_ratio=0.01  mu_visc_BF=[0, 0] N*m/(rad/s)  mu_visc=fs.mu_visc_tors N*m/(rad/s)  initial_deflection=0 rad  initial_velocity=0 rpm  num_supports=sdl.enum.num_supports.four  z_support=fs.z_support m  boundaryB1=sdl.enum.shaftSupport.bearingMatrix_speed  DrotB1_row=fs.bearing.d_rot N*m/(rad/s)  DtransB1_row=[20000, -44000, -44000, 350000] N/(m/s)  DtransB1_w_mat=fs.bearing.D N/(m/s)  KrotB1_row=fs.bearing.k_rot N*m/rad  KtransB1_row=[1000000, -200000, -300000, 5000000] N/m  KtransB1_w_mat=fs.bearing.K N/m  boundaryI1=sdl.enum.shaftSupport.bearingMatrix_speed  DrotI1_row=fs.bearing.d_rot N*m/(rad/s)  DtransI1_row=[20000, -44000, -44000, 350000] N/(m/s)  DtransI1_w_mat=fs.bearing.D N/(m/s)  KrotI1_row=fs.bearing.k_rot N*m/rad  KtransI1_row=[1000000, -200000, -300000, 5000000] N/m  KtransI1_w_mat=fs.bearing.K N/m  boundaryI2=sdl.enum.shaftSupport.bearingMatrix_speed  DrotI2_row=fs.bearing.d_rot N*m/(rad/s)  DtransI2_row=[20000, -44000, -44000, 350000] N/(m/s)  DtransI2_w_mat=fs.bearing.D N/(m/s)  KrotI2_row=fs.bearing.k_rot N*m/rad  KtransI2_row=[1000000, -200000, -300000, 5000000] N/m  KtransI2_w_mat=fs.bearing.K N/m  boundaryF1=sdl.enum.shaftSupport.bearingMatrix_speed  DrotF1_row=fs.bearing.d_rot N*m/(rad/s)  DtransF1_row=[20000, -44000, -44000, 350000] N/(m/s)  DtransF1_w_mat=fs.bearing.D N/(m/s)  KrotF1_row=fs.bearing.k_rot N*m/rad  KtransF1_row=[1000000, -200000, -300000, 5000000] N/m  KtransF1_w_mat=fs.bearing.K N/m  bearing_speed=fs.bearing_speed*fs.excitationPoles rpm  alpha=fs.a_damp 1/s  beta=fs.b_damp s  noDisk=sdl.enum.shaftDisks.disk  zDisk=fs.z_mass m  mDiskIN=fs.point_mass kg  IdDiskIN=fs.Id kg*m^2  IpDiskIN=fs.Ip./fs.excitationPoles kg*m^2  enable_static_unbalance=true  offsetMR=fs.excitationLoad./(fs.excitationPoles*fs.wNominal_forcing)^2 kg*m  offsetMR_initialAngleIN=0 rad  offsetMassLocation=fs.z_generator m  enable_external_force=false  externalForce=[1, 2] N  externalForceHarmonic=[.5, 2]  externalLoadAngle=[pi / 2, 3 * pi / 4] rad  zExternalLoad=[.25, .75] m  AnalysisMethod=sdl.enum.bendingAnalysisMethod.LumpedMass  ModeInputMethod=sdl.enum.modeInputMethod.SimscapeDetermined  numModesIn=fs.num_modes  mode_speed_dependency=sdl.enum.mode_speed_dependency.Dynamic  OmegaNom=fs.w_shaft_nominal rad/s  wMax=fs.wMax rad/s  dz=fs.dz m  userMode_w=[280, 644, 615, 1285] rad/s  userMode_w_mat=[257, 780, 580, 1560; 280, 644, 615, 1285; 294, 513, 636, 1020] rad/s  userMode_z=[0, .1, .2, .3, .4, .5, .6, .7, .8, .9, 1] m  userMode_shapeX=[.1648, .0086, -.2759, .0162; .1671, .0093, -.2231, .0133; .1691, .01, -.1689, .0102; .1707, .0105, -.1135, .007; .1717, .0108, -.057, .0035; .1721, .0109, 0, 0; .1717, .0108, .057, -.0035; .1707, .0105, .1135, -.007; .1691, .01, .1689, -.0102; .1671, .0093, .2231, -.0133; .1648, .0086, .2759, -.0162]  userMode_shapeX_mat=cat(3, [.1842, .0134, -.3072, .0272; .1863, .0152, -.2482, .0226; .1882, .0169, -.1878, .0176; .1897, .0182, -.1261, .0121; .1906, .019, -.0634, .0062; .191, .0193, 0, 0; .1906, .019, .0634, -.0062; .1897, .0182, .1261, -.0121; .1882, .0169, .1878, -.0176; .1863, .0152, .2482, -.0226; .1842, .0134, .3072, -.0272], [.1648, .0086, -.2759, .0162; .1671, .0093, -.2231, .0133; .1691, .01, -.1689, .0102; .1707, .0105, -.1135, .007; .1717, .0108, -.057, .0035; .1721, .0109, 0, 0; .1717, .0108, .057, -.0035; .1707, .0105, .1135, -.007; .1691, .01, .1689, -.0102; .1671, .0093, .2231, -.0133; .1648, .0086, .2759, -.0162], [.1291, .0046, -.2166, .0082; .131, .0048, -.1751, .0067; .1327, .005, -.1327, .0051; .1341, .0052, -.0891, .0035; .135, .0053, -.0448, .0017; .1353, .0053, 0, 0; .135, .0053, .0448, -.0017; .1341, .0052, .0891, -.0035; .1327, .005, .1327, -.0051; .131, .0048, .1751, -.0067; .1291, .0046, .2166, -.0082])  userMode_shapeY=[.1193, -.1784, -.1997, -.3348; .1209, -.1933, -.1615, -.2751; .1224, -.2068, -.1223, -.2119; .1235, -.2176, -.0821, -.1445; .1243, -.2245, -.0413, -.0734; .1246, -.2269, 0, 0; .1243, -.2245, .0413, .0734; .1235, -.2176, .0821, .1445; .1224, -.2068, .1223, .2119; .1209, -.1933, .1615, .2751; .1193, -.1784, .1997, .3348]  userMode_shapeY_mat=cat(3, [.0885, -.1625, -.1475, -.3301; .0895, -.1847, -.1192, -.2745; .0904, -.2048, -.0902, -.2141; .0911, -.2209, -.0606, -.1475; .0916, -.2313, -.0304, -.0754; .0917, -.2349, 0, 0; .0916, -.2313, .0304, .0754; .0911, -.2209, .0606, .1475; .0904, -.2048, .0902, .2141; .0895, -.1847, .1192, .2745; .0885, -.1625, .1475, .3301], [.1193, -.1784, -.1997, -.3348; .1209, -.1933, -.1615, -.2751; .1224, -.2068, -.1223, -.2119; .1235, -.2176, -.0821, -.1445; .1243, -.2245, -.0413, -.0734; .1246, -.2269, 0, 0; .1243, -.2245, .0413, .0734; .1235, -.2176, .0821, .1445; .1224, -.2068, .1223, .2119; .1209, -.1933, .1615, .2751; .1193, -.1784, .1997, .3348], [.1566, -.1901, -.2628, -.3377; .1589, -.1994, -.2125, -.2753; .161, -.2079, -.1609, -.2103; .1627, -.2146, -.1081, -.1424; .1638, -.219, -.0544, -.0719; .1642, -.2205, 0, 0; .1638, -.219, .0544, .0719; .1627, -.2146, .1081, .1424; .161, -.2079, .1609, .2103; .1589, -.1994, .2125, .2753; .1566, -.1901, .2628, .3377])  eta_lumped_nominal=1  etaDer_lumped_nominal=1  eta_modal_nominal=1  etaDer_modal_nominal=1
      settings: CopyFcn=simscape.engine.sli.internal.componentblockcallback(gcbh,'COPY')  PreCopyFcn=simscape.engine.sli.internal.componentblockcallback(gcbh,'PRECOPY')  PreDeleteFcn=simscape.engine.sli.internal.componentblockcallback(gcbh,'PREDELETE')  InternalSimscapePortConfiguration="{\"Bottom\":[],\"Left\":[{\"id\":\"B\",\"label\":\"B\",\"type\":\"foundation.mechanical.rotational.rotational\"}],\"Right\":[{\"id\":\"F\",\"label\":\"F\",\"type\":\"foundation.mechanical.rotational.rotational\"}],\"Top\":[]}"
      mask Type: Flexible Shaft
  B : PMIOPort  Side=Left
  G : PMIOPort  Port=2  Side=Left
  F : PMIOPort  Port=3  Side=Right
  connections:
  G/RConn1 -- Rigid Shaft Inertia/LConn1 -- F/RConn1
  Ideal Rotational Motion Sensor/RConn1 -- Ideal Angular Velocity Source/RConn2 -- Mechanical Rotational Reference/LConn1
  Rigid Shaft Inertia/RConn1 -- Ideal Rotational Motion Sensor/LConn1 -- B/RConn1
  Ideal Rotational Motion Sensor/RConn2 -- PS Gain/LConn1
  PS Gain/RConn1 -- Ideal Angular Velocity Source/RConn1
  Rotational Free End/LConn1 -- Torsion Dynamics/RConn1 -- Flexible Shaft Dynamics/RConn1
  Flexible Shaft Dynamics/LConn1 -- Ideal Angular Velocity Source/LConn1 -- Torsion Dynamics/LConn1
